simulink model "zad2"  (R2018a)
settings: Solver=VariableStepAuto  StartTime=0.0  StopTime=200  RelTol=1e-3
values from neighbouring files (symbols this model uses):
  Ke = Ke + K(1,i)    [Zad1a.m]    (also in Zad1b.m; Zad1c.m)
undefined symbols (not defined in the file or in its folder): Ku
settings Model: Creator=Szwank  LastModifiedBy=Szwank

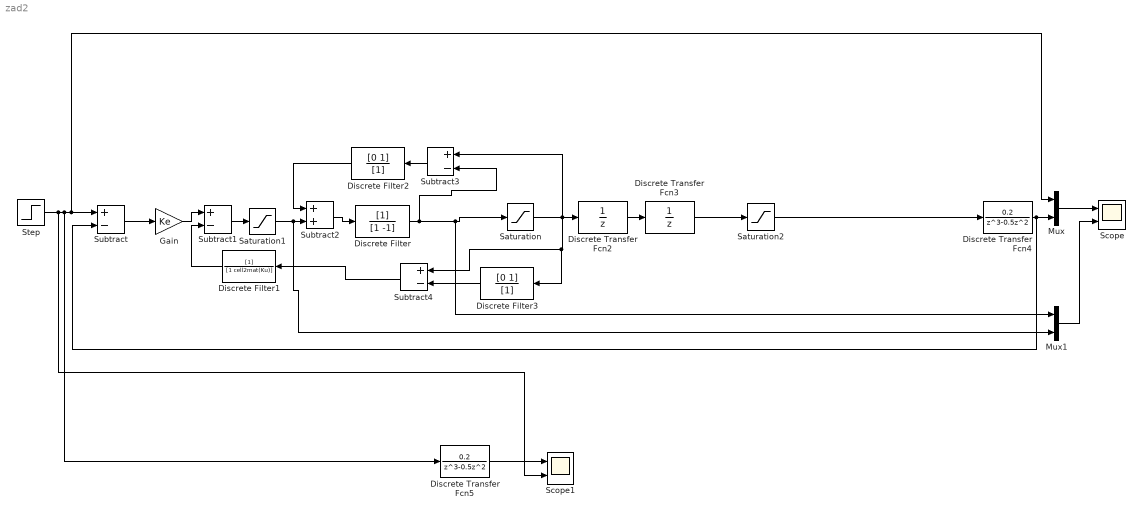
== system zad2 ==
  Discrete Transfer Fcn2 : DiscreteTransferFcn  Denominator=[1 0]
  Discrete Transfer Fcn3 : DiscreteTransferFcn  Denominator=[1 0]
  Discrete Transfer Fcn4 : DiscreteTransferFcn  Numerator=[0.2]  Denominator=[1 -0.5 0 0]  SampleTime=1
  Discrete Transfer Fcn5 : DiscreteTransferFcn  Numerator=[0.2]  Denominator=[1 -0.5 0 0]  SampleTime=1
  Discrete Filter : DiscreteFilter  Denominator=[1 -1]
  Discrete Filter1 : DiscreteFilter  Denominator=[1 cell2mat(Ku)]
  Discrete Filter2 : DiscreteFilter  Numerator=[0 1]  Denominator=[1]
  Discrete Filter3 : DiscreteFilter  Numerator=[0 1]  Denominator=[1]
  Gain : Gain  Gain=Ke
  Mux : Mux  Inputs=2
  Mux1 : Mux  Inputs=2
  Saturation : Saturate  UpperLimit=2.5  LowerLimit=-3
  Saturation1 : Saturate  UpperLimit=0.1  LowerLimit=-0.1
  Saturation2 : Saturate  UpperLimit=3  LowerLimit=-3
  Scope : Scope  NumInputPorts=2
  Scope1 : Scope  NumInputPorts=2
  Step : Step  SampleTime=0
  Subtract{,1,3..4} (4 alike) : Sum  Inputs=+-
  Subtract2 : Sum
  wires:
  Step/1 -> Scope1/2, Discrete Transfer Fcn5/1, Mux/1, Subtract/1
  Mux/1 -> Scope/1
  Mux1/1 -> Scope/2
  Discrete Transfer Fcn5/1 -> Scope1/1
  Discrete Transfer Fcn4/1 -> Subtract/2, Mux/2
  Subtract/1 -> Gain/1
  Discrete Transfer Fcn2/1 -> Discrete Transfer Fcn3/1
  Gain/1 -> Subtract1/1
  Discrete Filter1/1 -> Subtract1/2
  Subtract2/1 -> Discrete Filter/1
  Discrete Filter2/1 -> Subtract2/1
  Subtract3/1 -> Discrete Filter2/1
  Discrete Filter/1 -> Saturation/1, Mux1/1, Subtract3/2
  Saturation/1 -> Discrete Filter3/1, Subtract4/1, Subtract3/1, Discrete Transfer Fcn2/1
  Subtract1/1 -> Saturation1/1
  Saturation1/1 -> Mux1/2, Subtract2/2
  Discrete Filter3/1 -> Subtract4/2
  Subtract4/1 -> Discrete Filter1/1
  Discrete Transfer Fcn3/1 -> Saturation2/1
  Saturation2/1 -> Discrete Transfer Fcn4/1
